simulink model "NARMA"  (R2025b)
settings: Solver=FixedStepAuto  StartTime=0.0  StopTime=20  FixedStep=0.25  RelTol=1e-3
values from neighbouring files (symbols this model uses):
  Ki = vars(1)    [NFIntegradorSintonizacion.m]    (also in PIDSintotinizacion.m = vars(2))
undefined symbols (not defined in the file or in its folder): Lambda
libraries: fuzblock x1, neural x1, slpidlib x1
settings Model: Creator=Alessandro  LastModifiedBy=Alessandro
settings RTWCC: GPUComputeCapability=3.5

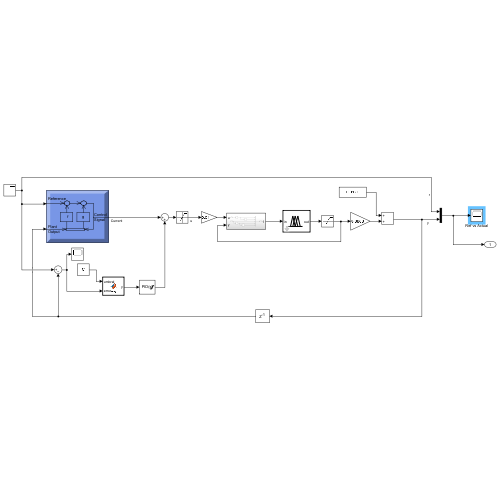
[thumbnail: Simulink's stored preview of the top-level diagram]
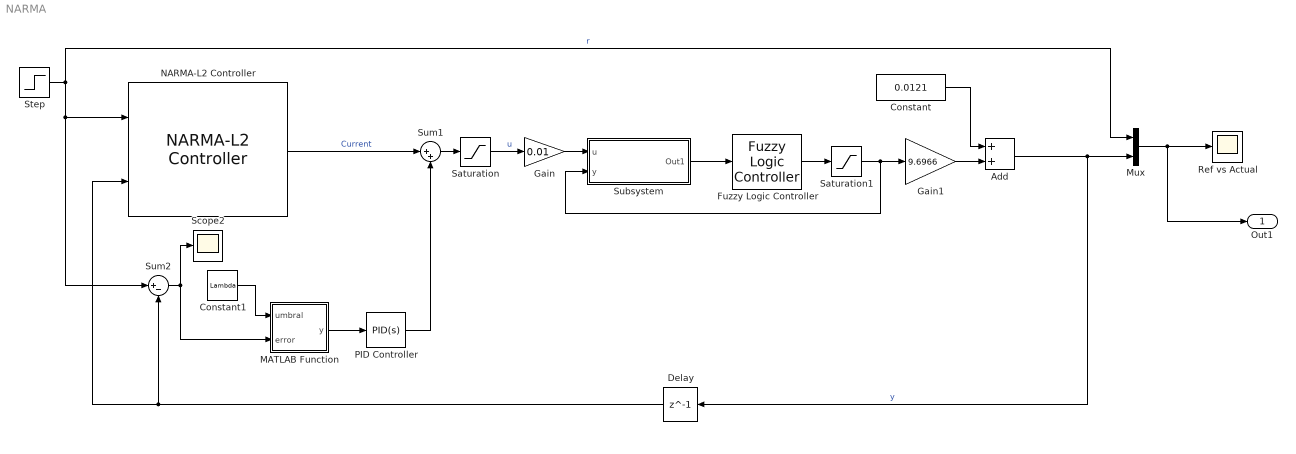
== system NARMA ==
  Add : Sum
  Constant : Constant  Value=0.0121
  Constant1 : Constant  Value=Lambda
  Delay : Delay  DelayLength=1
  Fuzzy Logic Controller : fuzblock/Fuzzy Logic  Controller  FIS='modelo_fr_dinamico.fis'  OutputSampleNumber=101  DataType=double  UseLookupTable=off  NumBreakpoints=10  FuzzifiedInputs=off  RuleFiringStrengths=off  RuleOutputs=off  AggregatedOutputs=off  SimulateUsing=Interpreted execution  OutOfRangeInputValueMessage=warning  NoRuleFiredMessage=warning  EmptyOutputFuzzySetMessage=warning
  Gain : Gain  Gain=0.01
  Gain1 : Gain  Gain=9.6966
  MATLAB Function : MATLAB Function  TreatAsAtomicUnit=on
  Mux : Mux  Inputs=2
  NARMA-L2 Controller : neural/Control Systems/NARMA-L2 Controller  Normalize=0  IW1_1=[-0.42467793216720606253 0.5692213355635036276;1.0777529613720591151 -1.486752018814940568;3.6389525259022832415 -7.1383142974827205052;-1.3230973726855641548 1.3397089782865698737;48.809347906680919493 -5.6664578363278756967]  IW3_2=[1.6215365077227488211 -7.2244624372244654609;0.5718477935160730663 -0.83782345745467867726;-4.8761260049301426989 11.035162408744922047;-0.052882865435311753044 -0.18674279984241015651;-0.50077741197961145314 0.23983466153446728053]  IW5_3=0.10775380693902895934  LW2_1=[-2.8824789717543368717 4.4995019497401012032 -1.7249143369849047058 -1.3989356243251251932 1.7615218513439732106]  LW4_3=[0.063416760414367639997 0.044127269503733933254 0.13379517768925641708 0.0035697472672307655785 0.01933019841866191052]  LW5_4=-0.38195262701407023398  LW6_5=0.31527802085501949181  LW6_2=0.010909076728393279909  B1=[-10.777248585611943099;4.7929874447760436595;-4.3831067075776202202;-11.043808207926202769;-22.913457224699410375]  B2=5.6967641046055916831  B3=[1.2566815093953946914;22.082130637635895454;-3.2967154719726496914;18.001519990091956913;-11.120556526666682373]  B4=-6.8614170778742584744  Limit_output=0  min_output=-Inf  max_output=Inf  Use_Previous_Weights=1  Ts=0.25  S1=5  Ni=1  Nj=2  sim_file=FT  trainfun=trainlm  Use_validation=1  Use_Testing=1  max_i=100  min_i=0  max_i_int=1  min_i_int=0.1  sam_training=1000  epochs=3000  minp=0.44840949110310884818  maxp=98.786848543652652666  mint=-0.2103463635115468966  maxt=98.786848543652652666
      link override Constant3: Value=Normalize
  PID Controller : slpidlib/PID Controller  Controller=PID  Form=Parallel  TimeDomain=Continuous-time  UseExternalTs=off  SampleTime=-1  IntegratorMethod=Forward Euler  FilterMethod=Forward Euler  ControllerParametersSource=internal  P=0  I=Ki  UseKiTs=off  D=0  UseExternalDerivativeSource=off  N=100  UseFilter=on  TunerSelectOption=Transfer Function Based (PID Tuner App)  InitialConditionSource=internal  InitialConditionForIntegrator=0  InitialConditionForFilter=0  DifferentiatorICPrevScaledInput=0  ExternalReset=none  TrackingMode=off  Kt=1  LimitOutput=on  SatLimitsSource=internal  UpperSaturationLimit=100  LowerSaturationLimit=-100  LinearizeAsGain=on  AntiWindupMode=none  Kb=1  LimitIntegrator=off  UpperIntegratorSaturationLimit=inf  LowerIntegratorSaturationLimit=-inf  POutMin=[]  POutMax=[]  IOutMin=[]  IOutMax=[]  DOutMin=[]  DOutMax=[]  NOutMin=[]  NOutMax=[]  SumOutMin=[]  SumOutMax=[]  SaturationOutMin=[]  SaturationOutMax=[]  PParamMin=[]  PParamMax=[]  IParamMin=[]  IParamMax=[]  DParamMin=[]  DParamMax=[]  NParamMin=[]  NParamMax=[]  KbParamMin=[]  KbParamMax=[]  KtParamMin=[]  KtParamMax=[]  KbOutMin=[]  KbOutMax=[]  KtOutMin=[]  KtOutMax=[]  IntegratorOutMin=[]  IntegratorOutMax=[]  FilterOutMin=[]  FilterOutMax=[]  SumI1OutMin=[]  SumI1OutMax=[]  SumI2OutMin=[]  SumI2OutMax=[]  SumI3OutMin=[]  SumI3OutMax=[]  SumI4OutMin=[]  SumI4OutMax=[]  SumDOutMin=[]  SumDOutMax=[]  DifferentiatorOutMin=[]  DifferentiatorOutMax=[]  FilterDiffOutCoefMin=[]  FilterDiffOutCoefMax=[]  ReciprocalOutMin=[]  ReciprocalOutMax=[]  SumDenOutMin=[]  SumDenOutMax=[]  SumNumOutMin=[]  SumNumOutMax=[]  DivideOutMin=[]  DivideOutMax=[]  UdiffTsProdOutMin=[]  UdiffTsProdOutMax=[]  NTsProdOutMin=[]  NTsProdOutMax=[]  UintegralTsProdOutMin=[]  UintegralTsProdOutMax=[]  UngainTsProdOutMin=[]  UngainTsProdOutMax=[]  ClampingZeroOutDataTypeStr=Inherit: Inherit via back propagation  ClampingZeroOutMin=[]  ClampingZeroOutMax=[]  FilterDenConstantOutDataTypeStr=Inherit: Inherit via back propagation  FilterDenConstantOutMin=[]  FilterDenConstantOutMax=[]  PCopyOutDataTypeStr=Inherit: Inherit via back propagation  PCopyOutMin=[]  PCopyOutMax=[]  NCopyOutDataTypeStr=Inherit: Inherit via back propagation  NCopyOutMin=[]  NCopyOutMax=[]  IntegratorContinuousStateAttributes=''  IntegratorStateMustResolveToSignalObject=off  IntegratorRTWStateStorageClass=Auto  FilterContinuousStateAttributes=''  FilterStateMustResolveToSignalObject=off  FilterRTWStateStorageClass=Auto  ParallelPVariant=InternalParameters  IdealPVariant=Disabled  IVariant=InternalParameters  DVariant=InternalParameters  IntegratorVariant=Continuous  SatVariant=Enabled  AWVariant=Passthrough  PCopyVariant=Disabled  TRVariant=Disabled  FdbkBlocksVariant=Forward  IdealPFdbkVariant=Disabled  SatFdbkVariant=Disabled  DerivativeFilterVariant=ContFilter  NVariant=InternalParameters  NCopyVariant=Disabled  FilterICVariant=InternalICsFilter  IntegratorICVariant=InternalICs  ExternalResetVariant=Disabled  TRSumVariant=Passthrough  SumFdbkVariant=Disabled  SumVariant=Sum_PID  TsampFilterVariant=InternalTs  TsampNgainVariant=Passthrough  TsampIntegralVariant=Disabled_SignalSpec  ExternalSaturationOutDataTypeStr=Inherit: Same as second input  DerivativeSourceVariant=ErrorSignal  PreIntVariant=InternalPreInt
  Ref vs Actual : Scope
      settings: ActiveDisplayYMinimum=5.217575511806845  ActiveDisplayYMaximum=8.1455172527195927  DataLoggingVariableName=Data_NARMA  DataLoggingSaveFormat=Array
  Saturation : Saturate  UpperLimit=100  LowerLimit=0
  Saturation1 : Saturate  UpperLimit=1  LowerLimit=0
  Scope2 : Scope
      settings: ActiveDisplayYMinimum=-1  ActiveDisplayYMaximum=1  DataLoggingVariableName=ScopeData3
  Step : Step  After=7  SampleTime=0
  Subsystem : Subsystem
  Sum1 : Sum  Inputs=|++
  Sum2 : Sum  Inputs=|+-
  Out1 : Outport
  wires:
  Gain1/1 -> Add/2
  Constant/1 -> Add/1
  Fuzzy Logic Controller/1 -> Saturation1/1
  Saturation1/1 -> Subsystem/2(y), Gain1/1
  Step/1 -> Mux/1, NARMA-L2 Controller/1, Sum2/1  "r"
  Mux/1 -> Out1/1, Ref vs Actual/1
  Delay/1 -> Sum2/2, NARMA-L2 Controller/2
  Add/1 -> Delay/1, Mux/2  "y"
  NARMA-L2 Controller/1 -> Sum1/1  "Current"
  Sum1/1 -> Saturation/1
  Sum2/1 -> MATLAB Function/2(error), Scope2/1
  Constant1/1 -> MATLAB Function/1(umbral)
  MATLAB Function/1(y) -> PID Controller/1
  PID Controller/1 -> Sum1/2
  Saturation/1 -> Gain/1  "u"
  Gain/1 -> Subsystem/1(u)
  Subsystem/1(Out1) -> Fuzzy Logic Controller/1

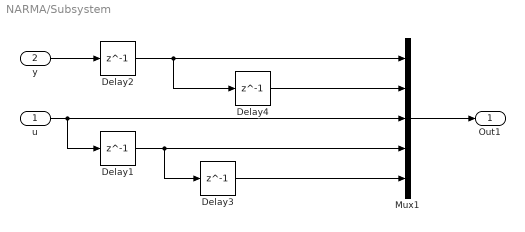
== system NARMA/Subsystem ==
  u : Inport
  y : Inport  Port=2
  Delay{1..4} (4 alike) : Delay  DelayLength=1
  Mux1 : Mux  Inputs=5
  Out1 : Outport
  wires:
  Mux1/1 -> Out1/1
  y/1 -> Delay2/1
  Delay2/1 -> Mux1/1, Delay4/1
  Delay4/1 -> Mux1/2
  u/1 -> Delay1/1, Mux1/3
  Delay3/1 -> Mux1/5
  Delay1/1 -> Delay3/1, Mux1/4

== matlab function NARMA/MATLAB Function ==
  data: umbral input; y output; error input
function y = fcn(umbral, error)
if (abs(error)<umbral)
    y = error;
else
    y = 0;
end
